simulink model "wenndlingfn"  (R2026a)
settings: Solver=ode45  StopTime=6
values from neighbouring files (symbols this model uses):
  A = 7    [wencode.m]
  B = 15    [wencode.m]
  G = 10    [wencode.m]
undefined symbols (not defined in the file or in its folder): a, b, C1, C2, C3, C4, C5, C6, C7, g
libraries: simulink x1
settings Model: Creator=acer  LastModifiedBy=acer

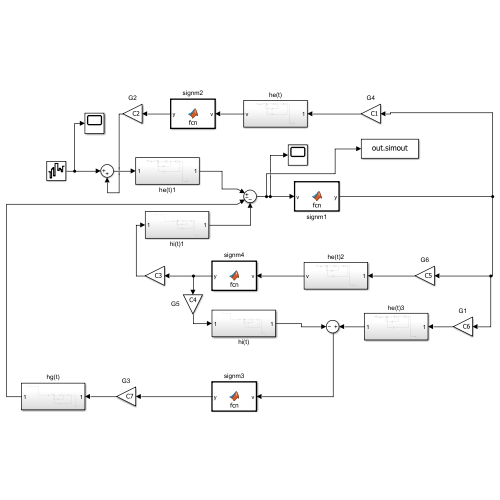
[thumbnail: Simulink's stored preview of the top-level diagram]
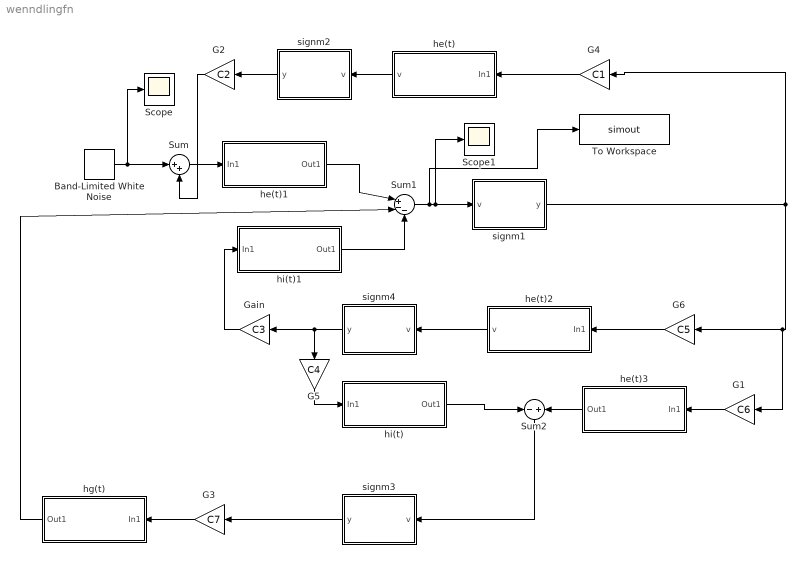
== system wenndlingfn ==
  Band-Limited White Noise : simulink/Sources/Band-Limited White Noise  Cov=[1]  Ts=0.001  seed=[23341]
  G1 : Gain  Gain=C6
  G2 : Gain  Gain=C2
  G3 : Gain  Gain=C7
  G4 : Gain  Gain=C1
  G5 : Gain  Gain=C4
  G6 : Gain  Gain=C5
  Gain : Gain  Gain=C3
  Scope : Scope
  Scope1 : Scope
      settings: ActiveDisplayYMinimum=-1  ActiveDisplayYMaximum=1
  Sum : Sum  Inputs=|++
  Sum1 : Sum  Inputs=|+--
  Sum2 : Sum  Inputs=-+
  To Workspace : ToWorkspace  VariableName=simout  SaveFormat=Timeseries  SampleTime=-1
  he(t) : Subsystem
  he(t)1 : Subsystem
  he(t)2 : Subsystem
  he(t)3 : Subsystem
  hg(t) : Subsystem
  hi(t) : Subsystem
  hi(t)1 : Subsystem
  signm1 : MATLAB Function  TreatAsAtomicUnit=on
  signm2 : MATLAB Function  TreatAsAtomicUnit=on
  signm3 : MATLAB Function  TreatAsAtomicUnit=on
  signm4 : MATLAB Function  TreatAsAtomicUnit=on
  wires:
  Band-Limited White Noise/1 -> Scope/1, Sum/1
  Sum/1 -> he(t)1/1(In1)
  G4/1 -> he(t)/1(In1)
  he(t)/1(v) -> signm2/1(v)
  signm2/1(y) -> G2/1
  G2/1 -> Sum/2
  he(t)1/1(Out1) -> Sum1/1
  Sum1/1 -> To Workspace/1, Scope1/1, signm1/1(v)
  signm1/1(y) -> G1/1, G6/1, G4/1
  hi(t)1/1(Out1) -> Sum1/3
  Gain/1 -> hi(t)1/1(In1)
  signm4/1(y) -> G5/1, Gain/1
  G5/1 -> hi(t)/1(In1)
  hi(t)/1(Out1) -> Sum2/1
  he(t)2/1(v) -> signm4/1(v)
  G6/1 -> he(t)2/1(In1)
  he(t)3/1(Out1) -> Sum2/2
  G1/1 -> he(t)3/1(In1)
  Sum2/1 -> signm3/1(v)
  signm3/1(y) -> G3/1
  G3/1 -> hg(t)/1(In1)
  hg(t)/1(Out1) -> Sum1/2

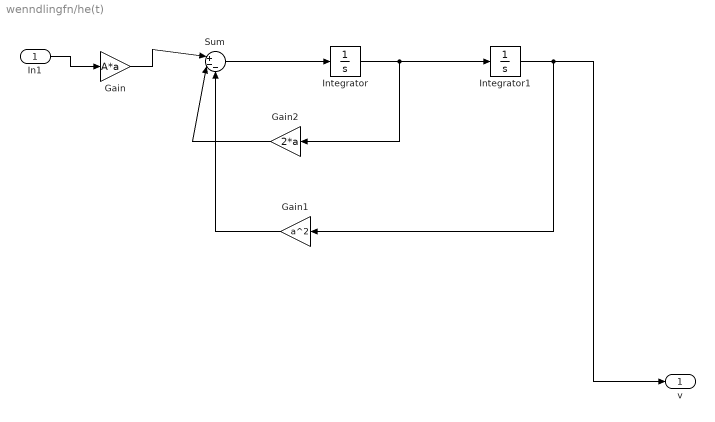
== system wenndlingfn/he(t) ==
  In1 : Inport
  Gain : Gain  Gain=A*a
  Gain1 : Gain  Gain=a^2
  Gain2 : Gain  Gain=2*a
  Integrator : Integrator
  Integrator1 : Integrator
  Sum : Sum  Inputs=|+--
  v : Outport
  wires:
  In1/1 -> Gain/1
  Gain/1 -> Sum/1
  Sum/1 -> Integrator/1
  Integrator/1 -> Gain2/1, Integrator1/1
  Integrator1/1 -> Gain1/1, v/1
  Gain2/1 -> Sum/2
  Gain1/1 -> Sum/3

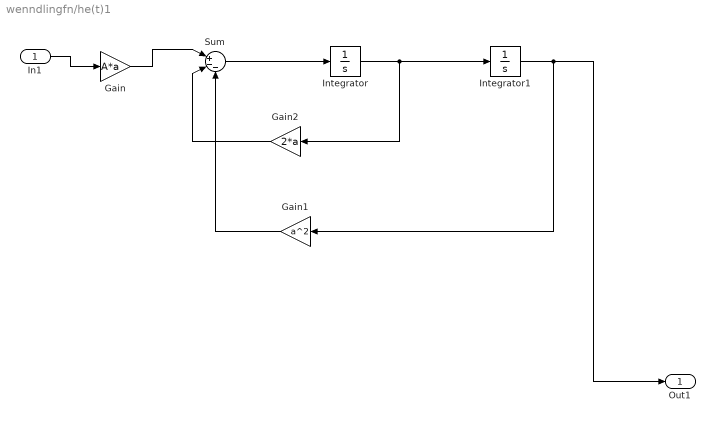
== system wenndlingfn/he(t)1 ==
  In1 : Inport
  Gain : Gain  Gain=A*a
  Gain1 : Gain  Gain=a^2
  Gain2 : Gain  Gain=2*a
  Integrator : Integrator
  Integrator1 : Integrator
  Sum : Sum  Inputs=|+--
  Out1 : Outport
  wires:
  In1/1 -> Gain/1
  Gain/1 -> Sum/1
  Sum/1 -> Integrator/1
  Integrator/1 -> Gain2/1, Integrator1/1
  Integrator1/1 -> Gain1/1, Out1/1
  Gain2/1 -> Sum/2
  Gain1/1 -> Sum/3

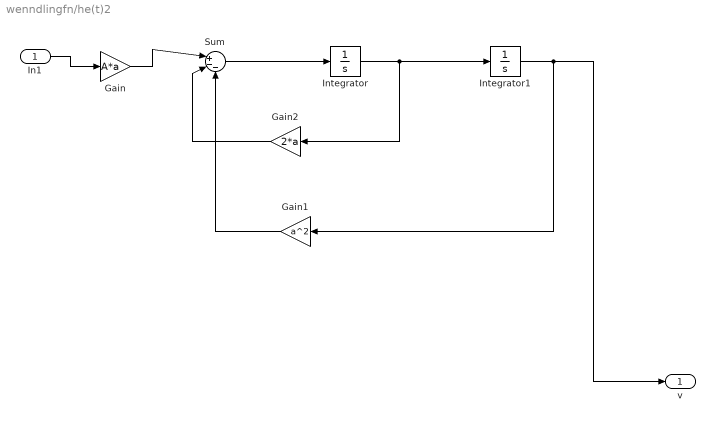
== system wenndlingfn/he(t)2 ==
  In1 : Inport
  Gain : Gain  Gain=A*a
  Gain1 : Gain  Gain=a^2
  Gain2 : Gain  Gain=2*a
  Integrator : Integrator
  Integrator1 : Integrator
  Sum : Sum  Inputs=|+--
  v : Outport
  wires:
  In1/1 -> Gain/1
  Gain/1 -> Sum/1
  Sum/1 -> Integrator/1
  Integrator/1 -> Gain2/1, Integrator1/1
  Integrator1/1 -> Gain1/1, v/1
  Gain2/1 -> Sum/2
  Gain1/1 -> Sum/3

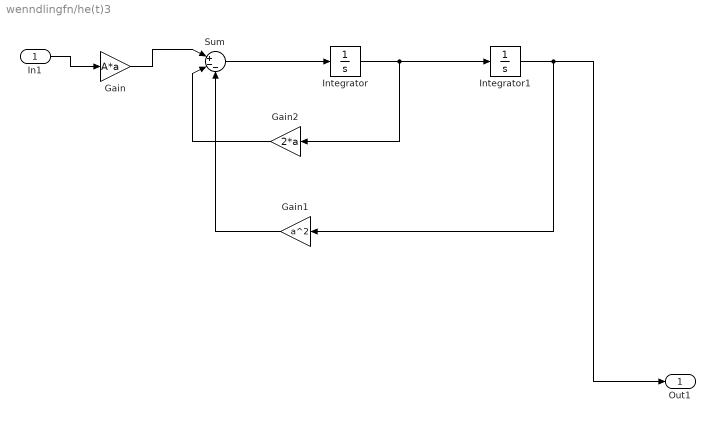
== system wenndlingfn/he(t)3 ==
  In1 : Inport
  Gain : Gain  Gain=A*a
  Gain1 : Gain  Gain=a^2
  Gain2 : Gain  Gain=2*a
  Integrator : Integrator
  Integrator1 : Integrator
  Sum : Sum  Inputs=|+--
  Out1 : Outport
  wires:
  In1/1 -> Gain/1
  Gain/1 -> Sum/1
  Sum/1 -> Integrator/1
  Integrator/1 -> Gain2/1, Integrator1/1
  Integrator1/1 -> Gain1/1, Out1/1
  Gain2/1 -> Sum/2
  Gain1/1 -> Sum/3

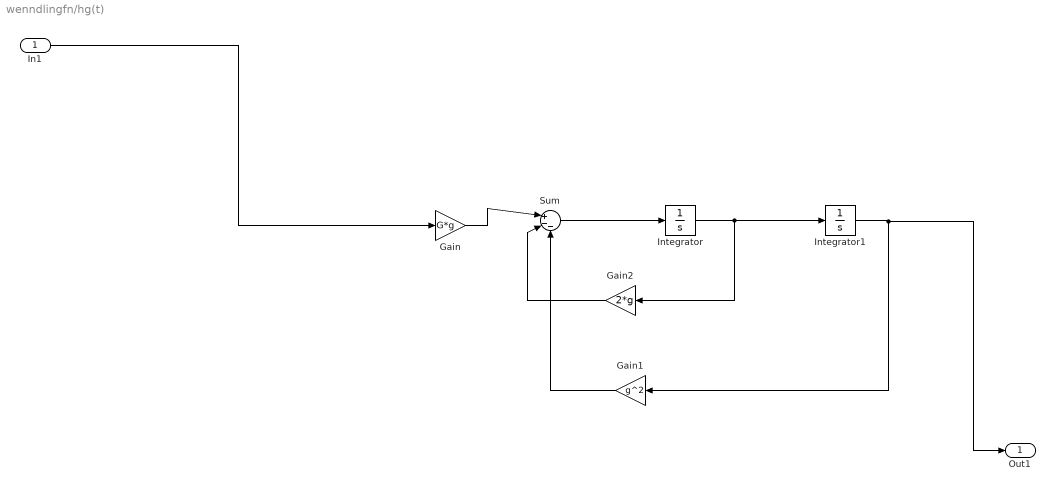
== system wenndlingfn/hg(t) ==
  In1 : Inport
  Gain : Gain  Gain=G*g
  Gain1 : Gain  Gain=g^2
  Gain2 : Gain  Gain=2*g
  Integrator : Integrator
  Integrator1 : Integrator
  Sum : Sum  Inputs=|+--
  Out1 : Outport
  wires:
  Integrator/1 -> Gain2/1, Integrator1/1
  Gain/1 -> Sum/1
  Sum/1 -> Integrator/1
  Gain2/1 -> Sum/2
  Gain1/1 -> Sum/3
  In1/1 -> Gain/1
  Integrator1/1 -> Out1/1, Gain1/1

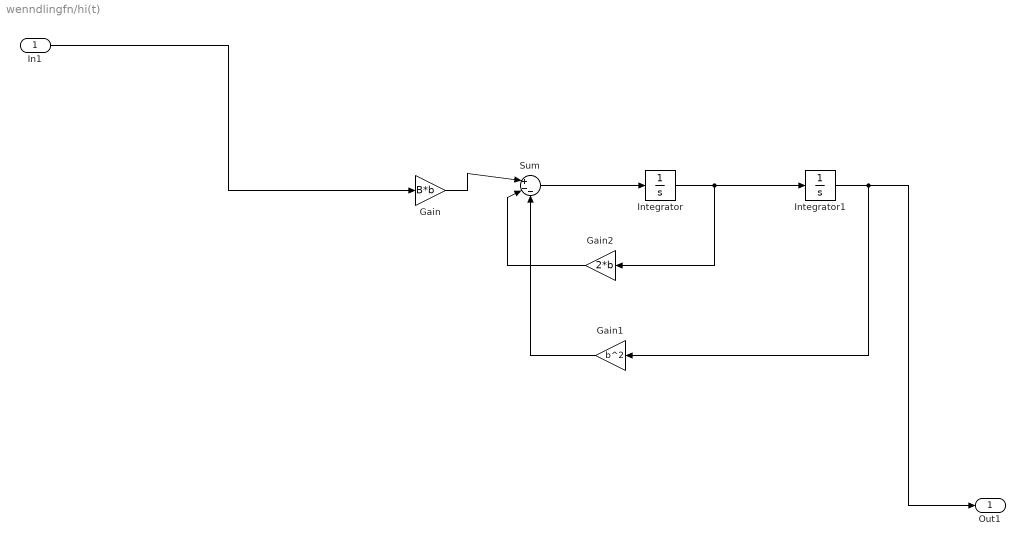
== system wenndlingfn/hi(t) ==
  In1 : Inport
  Gain : Gain  Gain=B*b
  Gain1 : Gain  Gain=b^2
  Gain2 : Gain  Gain=2*b
  Integrator : Integrator
  Integrator1 : Integrator
  Sum : Sum  Inputs=|+--
  Out1 : Outport
  wires:
  Integrator/1 -> Integrator1/1, Gain2/1
  Gain/1 -> Sum/1
  Integrator1/1 -> Out1/1, Gain1/1
  Sum/1 -> Integrator/1
  Gain2/1 -> Sum/2
  Gain1/1 -> Sum/3
  In1/1 -> Gain/1

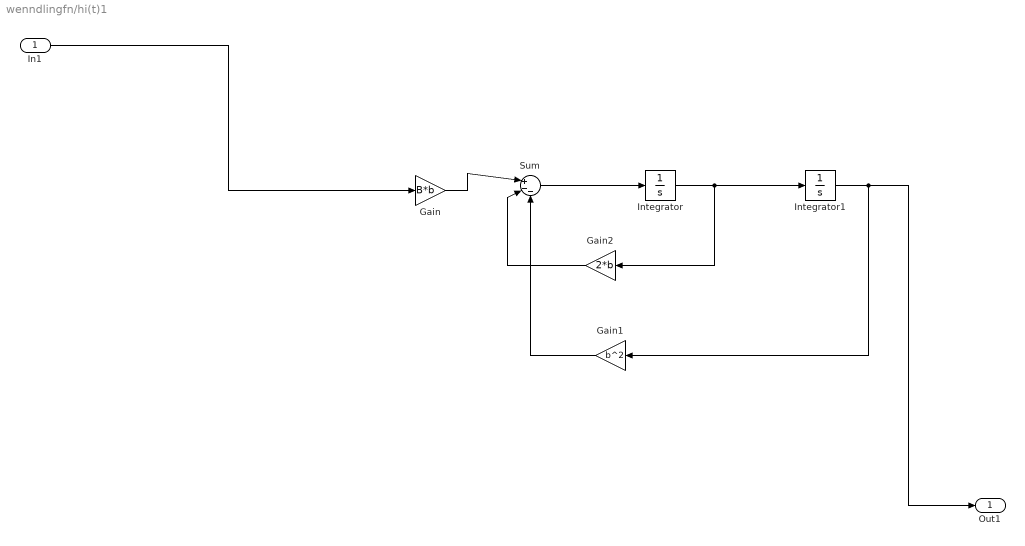
== system wenndlingfn/hi(t)1 ==
  In1 : Inport
  Gain : Gain  Gain=B*b
  Gain1 : Gain  Gain=b^2
  Gain2 : Gain  Gain=2*b
  Integrator : Integrator
  Integrator1 : Integrator
  Sum : Sum  Inputs=|+--
  Out1 : Outport
  wires:
  Integrator/1 -> Integrator1/1, Gain2/1
  Gain/1 -> Sum/1
  Integrator1/1 -> Out1/1, Gain1/1
  Sum/1 -> Integrator/1
  Gain2/1 -> Sum/2
  Gain1/1 -> Sum/3
  In1/1 -> Gain/1

== matlab function wenndlingfn/signm1 ==
  data: v input; y output
function y=fcn(v)

e0=2.5;
v0=6;
r=0.56;

y=(2*e0)/(1+exp(r*(v0-v)));

end

== matlab function wenndlingfn/signm3 ==
  data: v input; y output
function y=fcn(v)

e0=2.5;
v0=6;
r=0.56;

y=(2*e0)/(1+exp(r*(v0-v)));

end

== matlab function wenndlingfn/signm4 ==
  data: v input; y output
function y=fcn(v)

e0=2.5;
v0=6;
r=0.56;

y=(2*e0)/(1+exp(r*(v0-v)));

end

== matlab function wenndlingfn/signm2 ==
  data: v input; y output
function y=fcn(v)

e0=2.5;
v0=6;
r=0.56;

y=(2*e0)/(1+exp(r*(v0-v)));

end
